simulink library "lib_Convection_Gnielinski"  (R2015a)
settings: Solver=ode45  StartTime=0.0  StopTime=10.0  RelTol=1e-3
libraries: simulink x4, lib_Convection_ColebrookCorr x1, lib_GenTools_MinMax x1
settings Model: Creator=jlkratz  LastModifiedBy=jlkratz

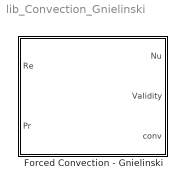
== system lib_Convection_Gnielinski ==
  Forced Convection - Gnielinski : Subsystem  mask(TSAT: Gnielinski's Correlation){SmoothOrRough_M=Rough, eoD_M=[0.02 0.01]}
      mask prompts: SmoothOrRough_M "SmoothOrRough_M - Check for a smooth surface, uncheck for a rough surface"; eoD_M "eoD_M - Relative roughness: surface roughness divided by the hydraulic diameter of the pipe (e/D)"
      mask help:
      | This block approximates the Nusselt number of a fully developed turbulent internal flow using Gnielinski's correlation. This block provides the option to consider a perfectly smooth or a rough surface. The user is cautioned that Gnielinski's correlation is valid for smooth tubes and so it may become less accurate as surface roughenss increases. Surface roughness is accounted for using the Colebrook correlation. The Colebrook correlation is solved using an iterative technique and so a convergence variable (conv) is output when this option is active so the it can be monitored. This correlaiton is valid for the following conditions:
      |
      | 0.5 <= Pr <= 2000
      | 3000 <= Re <= 5000000
      |
      | If any of these conditions are not met then the Validty output will be 1, otherwise it will be 0. In addition to these conditions one should keep in mind that this approximation is only valid for fully developed turbulent flow which is generally applicable when the flow is downstream of the inlet by a distance that is greater than or equal to 10 times the diamter of the tube (L/D >= 10).
      mask init:
      | % outport and constant block swapping -------------------------------------%
      | 
      | % Outport Numbers
      | n = 3; %first inport number
      | 
      | % Colebrook correlation convergence outport (conv)
      | if SmoothOrRough_M == 2
      |     if strcmp(get_param([gcb '/conv'],'BlockType'),'Terminator')
      |         MSK_ReplaceBlock_TSAT([gcb '/conv'],'built-in/Outport');
      |     end
      |     set_param([gcb '/conv'],'Port',num2str(n));
      |     n = n + 1;
      | else
      |     if strcmp(get_param([gcb '/conv'],'BlockType'),'Outport')
      |         MSK_ReplaceBlock_TSAT([gcb '/conv'],'built-in/Terminator');
      |         %set_param([gcb '/conv'],'Value','1');
      |     end
      | end
      mask Help: web(which('Convection_TSAT_Gnielinski.html'),'-helpbrowser')
      mask TypeOptions SmoothOrRough_M: Smooth | Rough
      mask Callback SmoothOrRough_M:
      | sel = get_param(gcb,'SmoothOrRough_M');
      | nobe = 'on';
      | if sel(1) == 'S'
      |     MSK_SEC_Enables3_TSAT('on',2,'dis')
      | elseif sel(1) == 'R'
      |     MSK_SEC_Enables3_TSAT('on',2,'en')
      | end
      | clear sel nobe

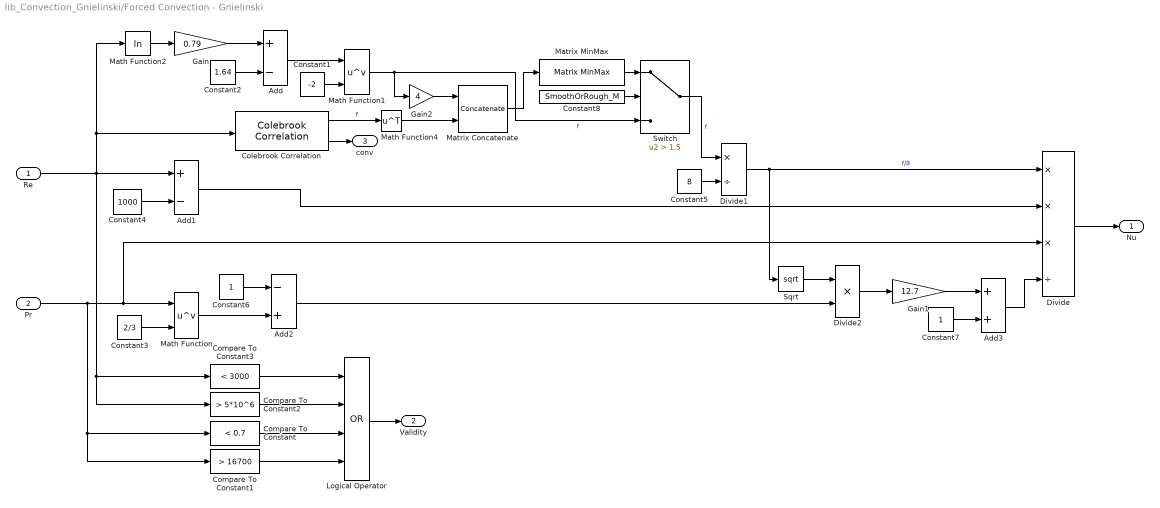
== system lib_Convection_Gnielinski/Forced Convection - Gnielinski ==
  Re : Inport
  Pr : Inport  Port=2
  Add : Sum  Inputs=+-
  Add1 : Sum  Inputs=+-
  Add2 : Sum  Inputs=-+
  Add3 : Sum
  Colebrook Correlation : lib_Convection_ColebrookCorr/Colebrook Correlation  eoD_M=eoD_M  BN_M=double(gcb)
  Compare To Constant : simulink/Logic and Bit Operations/Compare To Constant  relop=<  const=0.7  OutDataTypeStr=boolean
  Compare To Constant1 : simulink/Logic and Bit Operations/Compare To Constant  relop=>  const=16700  OutDataTypeStr=boolean
  Compare To Constant2 : simulink/Logic and Bit Operations/Compare To Constant  relop=>  const=5*10^6  OutDataTypeStr=boolean
  Compare To Constant3 : simulink/Logic and Bit Operations/Compare To Constant  relop=<  const=3000  OutDataTypeStr=boolean
  Constant1 : Constant  Value=-2
  Constant2 : Constant  Value=1.64
  Constant3 : Constant  Value=2/3
  Constant4 : Constant  Value=1000
  Constant5 : Constant  Value=8
  Constant6 : Constant
  Constant7 : Constant
  Constant8 : Constant  Value=SmoothOrRough_M
  Divide : Product  Inputs=***/
  Divide1 : Product  Inputs=*/
  Divide2 : Product  Inputs=**
  Gain : Gain  Gain=0.79
  Gain1 : Gain  Gain=12.7
  Gain2 : Gain  Gain=4
  Logical Operator : Logic  Operator=OR  Inputs=4  AllPortsSameDT=off  OutDataTypeStr=boolean
  Math Function : Math  Operator=pow  SaturateOnIntegerOverflow=on
  Math Function1 : Math  Operator=pow  SaturateOnIntegerOverflow=on
  Math Function2 : Math  Operator=log  SaturateOnIntegerOverflow=on
  Math Function4 : Math  Operator=transpose  SaturateOnIntegerOverflow=on
  Matrix Concatenate : Concatenate  Mode=Multidimensional array  ConcatenateDimension=2
  Matrix MinMax : lib_GenTools_MinMax/Matrix MinMax  rows_M=on  cols_M=off  all_M=off  minmax_M=on  BN_M=gcb
  Sqrt : Sqrt  SaturateOnIntegerOverflow=on
  Switch : Switch  Criteria=u2 > Threshold  Threshold=1.5
  Nu : Outport
  Validity : Outport  Port=2
  conv : Outport  Port=3
  wires:
  Math Function4/1 -> Matrix Concatenate/2
  Matrix MinMax/1 -> Switch/1
  Matrix Concatenate/1 -> Matrix MinMax/1
  Colebrook Correlation/1 -> Math Function4/1  "f"
  Gain2/1 -> Matrix Concatenate/1
  Colebrook Correlation/2 -> conv/1
  Switch/1 -> Divide1/1  "f"
  Math Function1/1 -> Switch/3, Gain2/1  "f"
  Add3/1 -> Divide/4
  Constant7/1 -> Add3/2
  Gain1/1 -> Add3/1
  Divide2/1 -> Gain1/1
  Add2/1 -> Divide2/2
  Sqrt/1 -> Divide2/1
  Constant6/1 -> Add2/1
  Math Function/1 -> Add2/2
  Divide/1 -> Nu/1
  Add1/1 -> Divide/2
  Divide1/1 -> Sqrt/1, Divide/1  "f/8"
  Constant5/1 -> Divide1/2
  Constant4/1 -> Add1/2
  Constant3/1 -> Math Function/2
  Constant1/1 -> Math Function1/2
  Add/1 -> Math Function1/1
  Constant2/1 -> Add/2
  Gain/1 -> Add/1
  Math Function2/1 -> Gain/1
  Compare To Constant3/1 -> Logical Operator/1
  Pr/1 -> Compare To Constant1/1, Compare To Constant/1, Math Function/1, Divide/3
  Re/1 -> Compare To Constant2/1, Compare To Constant3/1, Colebrook Correlation/1, Math Function2/1, Add1/1
  Compare To Constant1/1 -> Logical Operator/4
  Logical Operator/1 -> Validity/1
  Compare To Constant/1 -> Logical Operator/3
  Compare To Constant2/1 -> Logical Operator/2
  Constant8/1 -> Switch/2
